simulink model "NON_LINEAR_MODEL"  (R2023b)
settings: Solver=VariableStepAuto  StartTime=0.0  StopTime=10.0  RelTol=1e-3
values from neighbouring files (symbols this model uses):
  c = 8    [solar_tracker_constants.m]
  d = 0.11055    [solar_tracker_constants.m]
  g = 9.81    [solar_tracker_constants.m]
  J = 25.5759    [solar_tracker_constants.m]
  ke = 0.00083    [solar_tracker_constants.m]
  kt = 4    [solar_tracker_constants.m]
  L = 5e-3    (= 0.005)    [solar_tracker_constants.m]
  m = 98.87    [solar_tracker_constants.m]
  R = 0.5    [solar_tracker_constants.m]
libraries: simulink x2
settings Model: Creator=tinas  LastModifiedBy=tinas

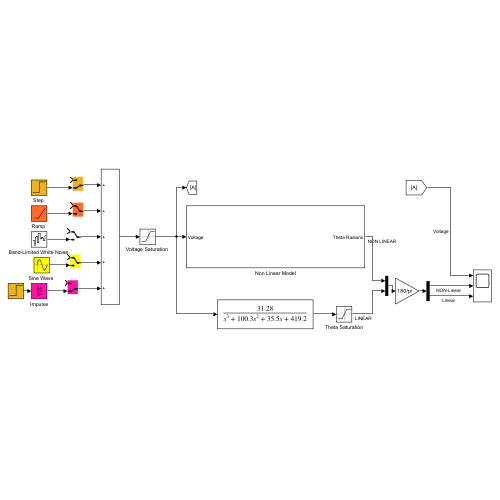
[thumbnail: Simulink's stored preview of the top-level diagram]
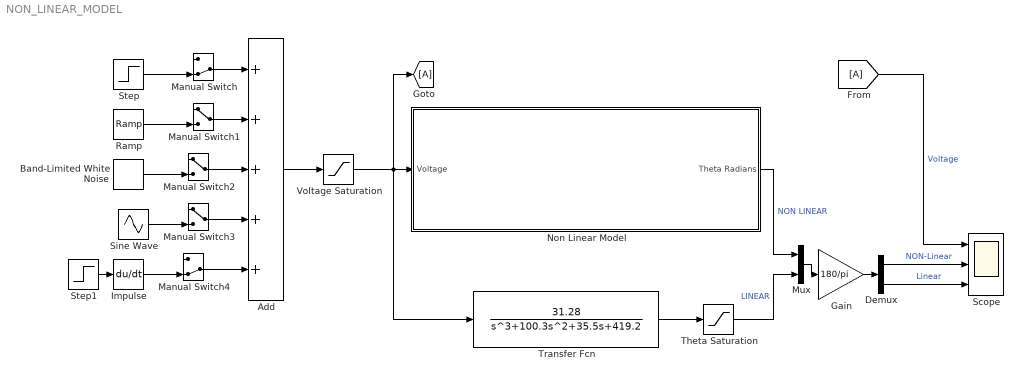
== system NON_LINEAR_MODEL ==
  Add : Sum  Inputs=+++++
  "Band-Limited White Noise " : simulink/Sources/Band-Limited White Noise  Cov=[0.1]  Ts=0.1  seed=[23341]
  Demux : Demux  Outputs=2
  From : From
  Gain : Gain  Gain=180/pi
  Goto : Goto
  Impulse : Derivative
  Manual Switch : ManualSwitch  CurrentSetting=0
  Manual Switch1 : ManualSwitch
  Manual Switch2 : ManualSwitch
  Manual Switch3 : ManualSwitch
  Manual Switch4 : ManualSwitch  CurrentSetting=0
  Mux : Mux  Inputs=2
  Non Linear Model : Subsystem
  "Ramp " : simulink/Sources/Ramp  slope=1  start=0  InitialOutput=0
  Scope : Scope  NumInputPorts=3
  "Sine Wave " : Sin  SampleTime=0
  "Step " : Step  After=100  SampleTime=0
  Step1 : Step  After=100  SampleTime=0
  Theta Saturation : Saturate  UpperLimit=pi/2  LowerLimit=-pi/2
  Transfer Fcn : TransferFcn  Numerator=[31.28]  Denominator="[1 100.3  35.5 419.2]"
  "Voltage Saturation " : Saturate  UpperLimit=230  LowerLimit=-230
  wires:
  Transfer Fcn/1 -> Theta Saturation/1
  "Voltage Saturation "/1 -> Transfer Fcn/1, Goto/1, Non Linear Model/1(Voltage)
  From/1 -> Scope/1  "Voltage"
  Add/1 -> "Voltage Saturation "/1
  Manual Switch/1 -> Add/1
  "Step "/1 -> Manual Switch/2
  Manual Switch1/1 -> Add/2
  "Ramp "/1 -> Manual Switch1/2
  Manual Switch2/1 -> Add/3
  "Band-Limited White Noise "/1 -> Manual Switch2/2
  Manual Switch3/1 -> Add/4
  "Sine Wave "/1 -> Manual Switch3/2
  Manual Switch4/1 -> Add/5
  Impulse/1 -> Manual Switch4/2
  Step1/1 -> Impulse/1
  Non Linear Model/1(Theta Radians) -> Mux/1  "NON LINEAR"
  Theta Saturation/1 -> Mux/2  "LINEAR"
  Mux/1 -> Gain/1
  Demux/1 -> Scope/2  "NON-Linear"
  Gain/1 -> Demux/1
  Demux/2 -> Scope/3  "Linear"

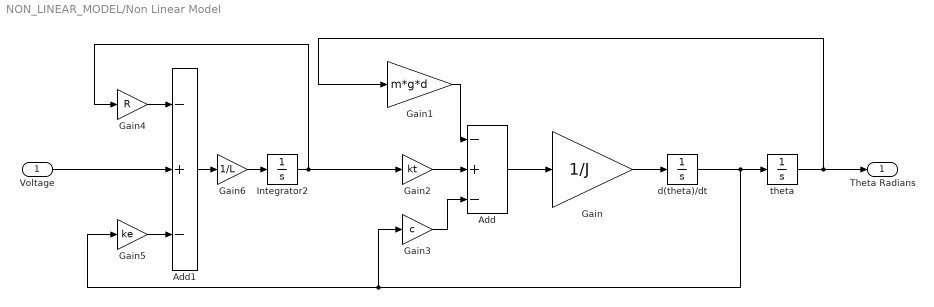
== system NON_LINEAR_MODEL/Non Linear Model ==
  Voltage : Inport
  Add : Sum  Inputs=-+-
  Add1 : Sum  Inputs=-+-
  Gain : Gain  Gain=1/J
  Gain1 : Gain  Gain=m*g*d
  Gain2 : Gain  Gain=kt
  Gain3 : Gain  Gain=c
  Gain4 : Gain  Gain=R
  Gain5 : Gain  Gain=ke
  Gain6 : Gain  Gain=1/L
  Integrator2 : Integrator
  d(theta)/dt : Integrator
  theta : Integrator  LimitOutput=on  UpperSaturationLimit=pi/2  LowerSaturationLimit=-pi/2
  Theta Radians : Outport
  wires:
  Gain2/1 -> Add/2
  Gain3/1 -> Add/3
  Gain5/1 -> Add1/3
  d(theta)/dt/1 -> theta/1, Gain5/1, Gain3/1
  Gain6/1 -> Integrator2/1
  Integrator2/1 -> Gain4/1, Gain2/1
  Gain/1 -> d(theta)/dt/1
  Voltage/1 -> Add1/2
  Add1/1 -> Gain6/1
  Gain4/1 -> Add1/1
  Add/1 -> Gain/1
  Gain1/1 -> Add/1
  theta/1 -> Gain1/1, Theta Radians/1
